simulink model "Lin_model_template_2015a"  (R2015a)
settings: Solver=ode45  SolverMode=SingleTasking  StartTime=0.0  StopTime=10.0  RelTol=1e-3
values from neighbouring files (symbols this model uses):
  a11 = -(C_f+C_r)/m*V    [Non_lin_template_mfile.m]
undefined symbols (not defined in the file or in its folder): a12, b11, b12, delta_f, delta_r
settings Model: CovMetricSettings=dwe  CovHtmlReporting=off  covSaveCumulativeToWorkspaceVar=off  CovSaveSingleToWorkspaceVar=off  CovExternalEMLEnable=on  Creator=Instructor  LastModifiedBy=Santo
settings DataIOCC: LimitDataPoints=off  SaveFormat=Dataset
settings DebuggingCC: SFUnexpectedBacktrackingDiag=error  SFNoUnconditionalDefaultTransitionDiag=error
settings HardwareCC: ProdBitPerPointer=64  ProdLargestAtomicFloat=Float  ProdIntDivRoundTo=Zero  ProdEndianess=LittleEndian  ProdHWDeviceType=Specified
settings ModelReferenceCC: PropagateSignalLabelsOutOfModel=on
settings GRTTargetCC: TargetLangStandard=C99 (ISO)  GeneratePreprocessorConditionals=Use local settings

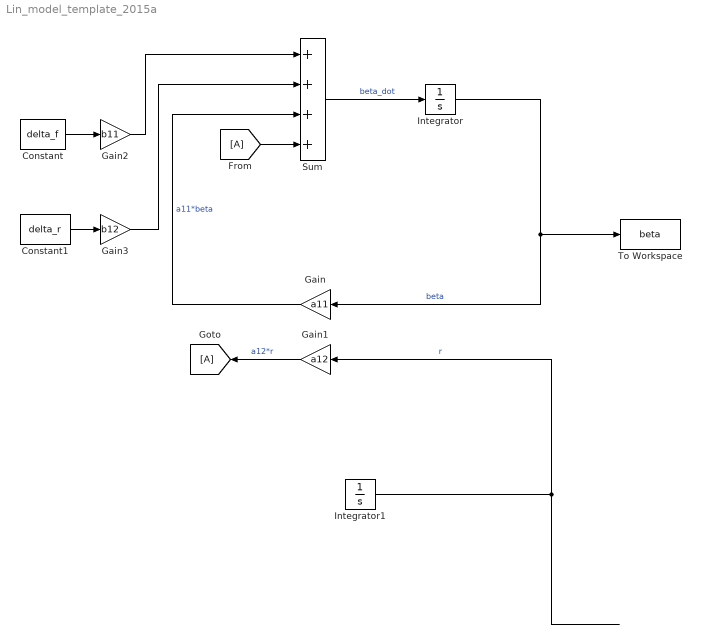
== system Lin_model_template_2015a ==
  Constant : Constant  Value=delta_f
  Constant1 : Constant  Value=delta_r
  Gain : Gain  Gain=a11
  Gain1 : Gain  Gain=a12
  Gain2 : Gain  Gain=b11
  Gain3 : Gain  Gain=b12
  Integrator : Integrator
  Integrator1 : Integrator
  Sum : Sum  Inputs=++++
  To Workspace : ToWorkspace  VariableName=beta  SaveFormat=Timeseries  SampleTime=-1
  wires:
  Integrator/1 -> To Workspace/1, Gain/1  "beta"
  Sum/1 -> Integrator/1  "beta_dot"
  ? -> Integrator1/1  "r_dot"
  Integrator1/1 -> Gain1/1  "r"
  Gain/1 -> Sum/3  "a11*beta"
  Gain1/1 -> [A]  "a12*r"
  Constant/1 -> Gain2/1
  Constant1/1 -> Gain3/1
  Gain2/1 -> Sum/1
  Gain3/1 -> Sum/2
  [A] -> Sum/4
